simulink model "HIL_FormationFlying"  (R2023a)
settings: Solver=FixedStepAuto  StartTime=0.0  StopTime=T1  FixedStep=dt  RelTol=1e-3
undefined symbols (not defined in the file or in its folder): r1_I_ini, r2_I_ini, v1_I_ini, v2_I_ini
libraries: slrealtimeiplib x1, instrumentseriallib x1
settings Model: Creator=Yazan  LastModifiedBy=Yazan
settings DataIOCC: SaveFormat=Array  ReturnWorkspaceOutputs=off
settings OptimizationCC: DefaultParameterBehavior=Inlined  EnhancedBackFolding=on  PassReuseOutputArgsAs=Individual arguments  ZeroExternalMemoryAtStartup=off  ZeroInternalMemoryAtStartup=off  MaxStackSize=64  OptimizeBlockOrder=speed  DifferentSizesBufferReuse=on  OptimizationCustomize=off  EfficientTunableParamExpr=on
settings DebuggingCC: ParameterTunabilityLossMsg=error  UnconnectedInputMsg=warning  UnconnectedOutputMsg=warning  UnconnectedLineMsg=warning
settings HardwareCC: ProdBitPerLong=64  ProdLargestAtomicInteger=LongLong  ProdLargestAtomicFloat=Double  ProdLongLongMode=on  ProdHWDeviceType=ARM Compatible->ARM 64-bit (LP64)
settings ModelReferenceCC: EnableRefExpFcnMdlSchedulingChecks=on
settings SFSimCC: MATLABDynamicMemAlloc=off
settings RTWCC: Description=Embedded Coder  SystemTargetFile=ert.tlc  TemplateMakefile=ert_default_tmf  DLArmComputeVersion=19.05
settings CodeAppCC: ForceParamTrailComments=on  IgnoreCustomStorageClasses=off  OperatorAnnotations=on  SimulinkDataObjDesc=on  SFDataObjDesc=on  InsertBlockDesc=on
settings ERTTargetCC: InlinedParameterPlacement=NonHierarchical  ERTCustomFileTemplate=example_file_process.tlc

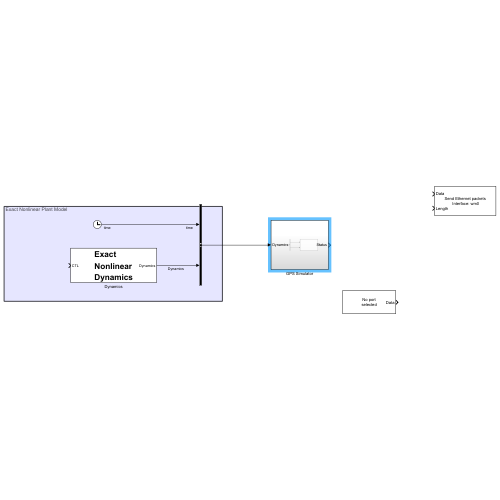
[thumbnail: Simulink's stored preview of the top-level diagram]
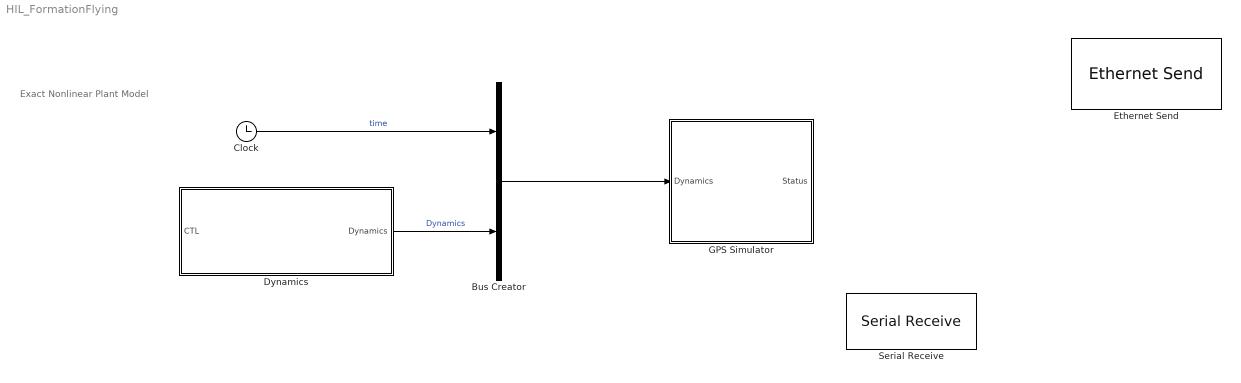
== system HIL_FormationFlying ==
  note: Exact Nonlinear Plant Model
  Bus Creator : BusCreator  Inputs=2
  Clock : Clock
  Dynamics : Subsystem
      mask Display: disp(['{\bf\fontsize{20}Exact}' newline newline '{\bf\fontsize{20}Nonlinear}' newline newline '{\bf\fontsize{20}Dynamics}'], 'texmode','on');
  Ethernet Send : slrealtimeiplib/Ethernet/Ethernet Send  InterfaceName=wm0  OverwriteSrcMACAddress=off  MessageIn=off  SampleTime=-1
  GPS Simulator : Subsystem  InitFcn=initialization
  Serial Receive : instrumentseriallib/Serial Receive  Priority=1  PortSel=<Select a port...>  Port=<Select a port...>  ComPort=<Select a port...>  DataType=uint8  SaveDataType=uint8  ToggleHeader=off  Header=[]  ToggleTerminator=off  Terminator=<none>  CustomTerminator=[]  InputFormat=Column major  ToggleDataSize=on  DataSize=[1 1]  EnableBlockingMode=on  ActionDataUnavailable=Output last received value  ActionWhenDataUnavailable=Output last received value  CustomValue=0  SampleTime=0.01  SimulateUsing=Interpreted execution  BlockInModel=on  aMode=1
  wires:
  Dynamics/1(Dynamics) -> Bus Creator/2  "Dynamics"
  Clock/1 -> Bus Creator/1  "time"
  Bus Creator/1 -> GPS Simulator/1(Dynamics)

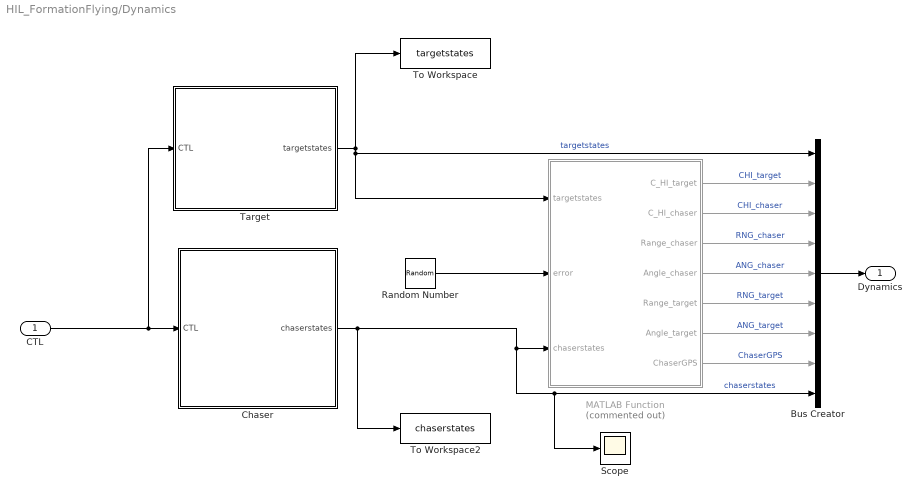
== system HIL_FormationFlying/Dynamics ==
  CTL : Inport
  Bus Creator : BusCreator  Inputs=9
  Chaser : Subsystem
  MATLAB Function : MATLAB Function  Commented=on  TreatAsAtomicUnit=on
  Random Number : RandomNumber  Mean=[0;0;0;0;0;0;0;0;0;0;0;0]  Variance=[10;0.00001;0.00001;10;0.00001;0.00001;0.001;0.001;0.001;0.0001;0.0001;0.0001]  Seed=[100;200;300;400;500;600;700;800;900;1000;1100;1200]  SampleTime=1
  Scope : Scope
  Target : Subsystem
  To Workspace : ToWorkspace  VariableName=targetstates  SampleTime=-1
  To Workspace2 : ToWorkspace  VariableName=chaserstates  SampleTime=-1
  Dynamics : Outport
  wires:
  Chaser/1(chaserstates) -> To Workspace2/1, Scope/1, Bus Creator/9, MATLAB Function/3(chaserstates)  "chaserstates"
  CTL/1 -> Target/1(CTL), Chaser/1(CTL)
  MATLAB Function/1(C_HI_target) -> Bus Creator/2  "CHI_target"
  MATLAB Function/2(C_HI_chaser) -> Bus Creator/3  "CHI_chaser"
  MATLAB Function/3(Range_chaser) -> Bus Creator/4  "RNG_chaser"
  MATLAB Function/4(Angle_chaser) -> Bus Creator/5  "ANG_chaser"
  MATLAB Function/5(Range_target) -> Bus Creator/6  "RNG_target"
  MATLAB Function/6(Angle_target) -> Bus Creator/7  "ANG_target"
  Bus Creator/1 -> Dynamics/1
  Target/1(targetstates) -> MATLAB Function/1(targetstates), Bus Creator/1, To Workspace/1  "targetstates"
  Random Number/1 -> MATLAB Function/2(error)
  MATLAB Function/7(ChaserGPS) -> Bus Creator/8  "ChaserGPS"

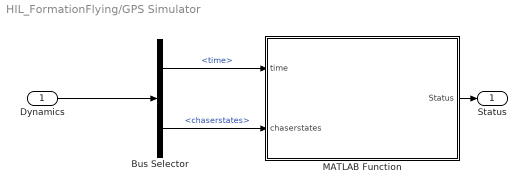
== system HIL_FormationFlying/GPS Simulator ==
  Dynamics : Inport
  Bus Selector : BusSelector  OutputSignals=time,Dynamics.chaserstates
  MATLAB Function : MATLAB Function  TreatAsAtomicUnit=on
  Status : Outport
  wires:
  Bus Selector/2 -> MATLAB Function/2(chaserstates)  "<chaserstates>"
  MATLAB Function/1(Status) -> Status/1
  Bus Selector/1 -> MATLAB Function/1(time)  "<time>"
  Dynamics/1 -> Bus Selector/1

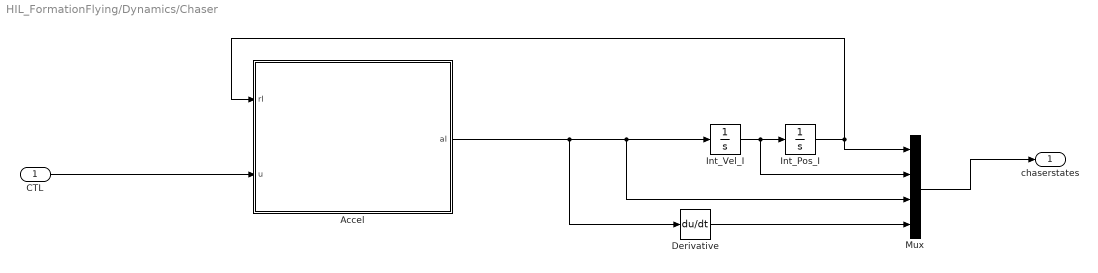
== system HIL_FormationFlying/Dynamics/Chaser ==
  CTL : Inport
  Accel : MATLAB Function  TreatAsAtomicUnit=on
  Derivative : Derivative
  Int_Pos_I : Integrator  InitialCondition=r2_I_ini
  Int_Vel_I : Integrator  InitialCondition=v2_I_ini
  Mux : Mux
  chaserstates : Outport
  wires:
  Int_Pos_I/1 -> Accel/1(rI), Mux/1
  Accel/1(aI) -> Derivative/1, Mux/3, Int_Vel_I/1
  Int_Vel_I/1 -> Mux/2, Int_Pos_I/1
  Mux/1 -> chaserstates/1
  CTL/1 -> Accel/2(u)
  Derivative/1 -> Mux/4

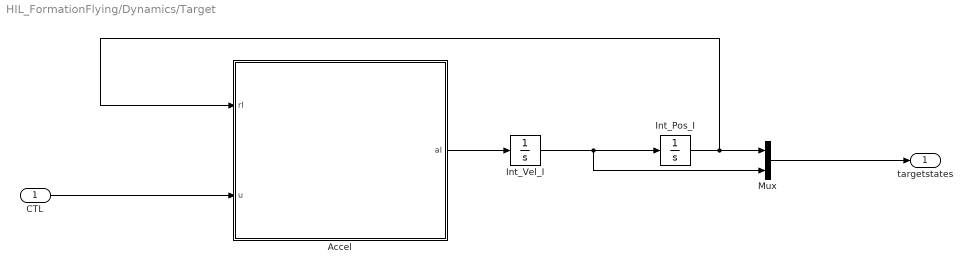
== system HIL_FormationFlying/Dynamics/Target ==
  CTL : Inport
  Accel : MATLAB Function  TreatAsAtomicUnit=on
  Int_Pos_I : Integrator  InitialCondition=r1_I_ini
  Int_Vel_I : Integrator  InitialCondition=v1_I_ini
  Mux : Mux  Inputs=2
  targetstates : Outport
  wires:
  Int_Pos_I/1 -> Mux/1, Accel/1(rI)
  Accel/1(aI) -> Int_Vel_I/1
  Int_Vel_I/1 -> Int_Pos_I/1, Mux/2
  Mux/1 -> targetstates/1
  CTL/1 -> Accel/2(u)

== matlab function HIL_FormationFlying/GPS Simulator/MATLAB Function ==
  data: Status output; time input; chaserstates input; t parameter
function Status  = SetSpacecraftPosition_GPSSIM(time,chaserstates, t)

end

== matlab function HIL_FormationFlying/Dynamics/Target/Accel ==
  data: rI input; u input; aI output
function aI  = Accel(rI,u)
aI = [0;0;0];
aI = aI + u;
r = sqrt(rI(1)^2 + rI(2)^2 + rI(3)^2);
mu_Earth   = 398600.4418;
aI = -mu_Earth/(r^3).*rI + aI;
end

== matlab function HIL_FormationFlying/Dynamics/Chaser/Accel ==
  data: rI input; u input; aI output
function aI  = Accel(rI,u)
aI = [0;0;0];
aI = aI + u;
r = sqrt(rI(1)^2 + rI(2)^2 + rI(3)^2);
mu_Earth   = 398600.4418;
aI = -mu_Earth/(r^3).*rI + aI;
end

== matlab function HIL_FormationFlying/Dynamics/MATLAB Function ==
  data: targetstates input; error input; C_HI_target output; chaserstates input; C_HI_chaser output; Range_chaser output; Angle_chaser output; Range_target output; Angle_target output; ChaserGPS output
function [C_HI_target,C_HI_chaser,Range_chaser,Angle_chaser,Range_target,Angle_target,ChaserGPS] = LVLH(targetstates,error, chaserstates)

C_HI_target = CHI(targetstates);
C_HI_chaser = CHI(chaserstates);
ChaserGPS = chaserstates + error(7:12);
RelPos_chaser = C_HI_chaser*(targetstates(1:3)-chaserstates(1:3)).*1000;
[RNG_chaser,ANG_chaser] = rangeangle(RelPos_chaser);
Range_chaser = RNG_chaser + error(1);
Az_chaser = ANG_chaser(1) + error(2);
El_chaser = ANG_chaser(2) + error(3);
% Range = sqrt(RelPos(1)^2 + RelPos(2)^2 + RelPos(3)^2);
% El = asin(RelPos(3)/Range)*180/pi;
% Az = asin(RelPos(2)/(Range*cos(El*pi/180)))*180/pi;
% Range = RangeCal(1,1);
% Az = AngleCal(1,1);
% El = AngleCal(2,1);
Angle_chaser = [Az_chaser;El_chaser];

RelPos_target = C_HI_target*(chaserstates(1:3)-targetstates(1:3)).*1000;
[RNG_target,ANG_target] = rangeangle(RelPos_target);
Range_target = RNG_target + error(4);
Az_target = ANG_target(1) + error(5);
El_target = ANG_target(2) + error(6);
% Range = sqrt(RelPos(1)^2 + RelPos(2)^2 + RelPos(3)^2);
% El = asin(RelPos(3)/Range)*180/pi;
% Az = asin(RelPos(2)/(Range*cos(El*pi/180)))*180/pi;
% Range = RangeCal(1,1);
% Az = AngleCal(1,1);
% El = AngleCal(2,1);
Angle_target = [Az_target;El_target];


end
function C_HI =  CHI(states)

% ---------------------------------------------------------------
% CHI
% ---------------------------------------------------------------
% Description:
% Compute the rotation matrix from ECI to Hill's, i.e. C_HI
% ---------------------------------------------------------------
% Inputs:
% r_I => components of r in ECI (3 x 1 matrix)
% v_I => components of v in ECI (3 x 1 matrix)
% ---------------------------------------------------------------
% Outputs:
% C_HI => rotation matrix from ECI to Hill's (3 x 3 matrix)
% ---------------------------------------------------------------
% Parameters:
% None
% ---------------------------------------------------------------
% Copyright:
% Steve Ulrich, 2015 
% ---------------------------------------------------------------
r_I = states(1:3);
v_I = states(4:6);
Hx = zeros(3,1);
Hy = zeros(3,1);
Hz = zeros(3,1);
C_HI = zeros(3);

% Compute orbital radius and orbital speed
rmod = sqrt(r_I(1)*r_I(1) + r_I(2)*r_I(2) + r_I(3)*r_I(3));
vmod = sqrt(v_I(1)*v_I(1) + v_I(2)*v_I(2) + v_I(3)*v_I(3));

% Compute Hx unit vector, i.e., first row of C_HI
Hx(1) = r_I(1)/rmod;
Hx(2) = r_I(2)/rmod;
Hx(3) = r_I(3)/rmod;

% Compute Hz unit vector, i.e., third row of C_HI
Hz(1) = (-Hx(3)*v_I(2)+Hx(2)*v_I(3));
Hz(2) = ( Hx(3)*v_I(1)-Hx(1)*v_I(3));
Hz(3) = (-Hx(2)*v_I(1)+Hx(1)*v_I(2));

Hzmod = sqrt(Hz(1)^2+Hz(2)^2+Hz(3)^2);

Hz(1) = Hz(1)/Hzmod;
Hz(2) = Hz(2)/Hzmod;
Hz(3) = Hz(3)/Hzmod;

% Compute Hy unit vector, i.e., second row of C_HI
Hy(1) = (-Hz(3)*Hx(2)+Hz(2)*Hx(3));
Hy(2) = ( Hz(3)*Hx(1)-Hz(1)*Hx(3));
Hy(3) = (-Hz(2)*Hx(1)+Hz(1)*Hx(2));

C_HI = [Hx(1), Hx(2), Hx(3); Hy(1), Hy(2), Hy(3); Hz(1), Hz(2), Hz(3)];


end
